simulink model "Laborki1_z2"  (R2017a)
settings: Solver=VariableStepAuto  StartTime=0.0  StopTime=10.0  RelTol=1e-3
settings Model: Creator=DoktorHax  LastModifiedBy=DoktorHax

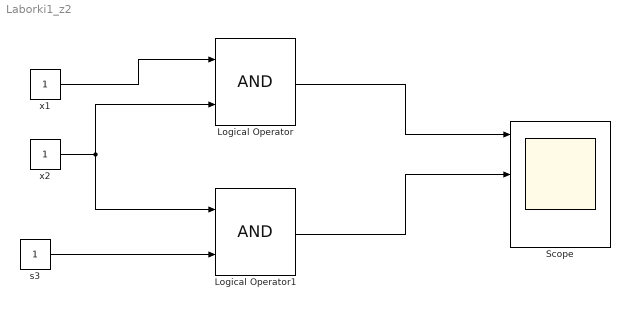
== system Laborki1_z2 ==
  Logical Operator : Logic  AllPortsSameDT=off  OutDataTypeStr=boolean
  Logical Operator1 : Logic  AllPortsSameDT=off  OutDataTypeStr=boolean
  Scope : Scope  NumInputPorts=6
  s3 : Constant
  x1 : Constant
  x2 : Constant
  wires:
  x1/1 -> Logical Operator/1
  x2/1 -> Logical Operator1/1, Logical Operator/2
  s3/1 -> Logical Operator1/2
  Logical Operator1/1 -> Scope/3
  Logical Operator/1 -> Scope/1
